simulink model "verify_Radiator_basic_mdl"  (R2016b)
settings: Solver=ode45  StartTime=0.0  StopTime=4800  MaxStep=100  RelTol=1e-3  EnableMultiTasking=on
undefined symbols (not defined in the file or in its folder): heat_capacity
libraries: carnot x2, simulink x1
settings Model: Creator=drhf  LastModifiedBy=drhf
settings DataIOCC: LimitDataPoints=on  SaveFormat=Array  SignalLoggingSaveFormat=ModelDataLogs
settings OptimizationCC: ExpressionDepthLimit=2147483647  LifeSpan=inf
settings DebuggingCC: UnderspecifiedInitializationDetection=Classic  MergeDetectMultiDrivingBlocksExec=none  SolverPrmCheckMsg=warning  FcnCallInpInsideContextMsg=warning  StateNameClashWarn=warning  SFUnexpectedBacktrackingDiag=warning  SFNoUnconditionalDefaultTransitionDiag=warning  SFExecutionAtInitializationDiag=none
settings HardwareCC: ProdBitPerPointer=32  ProdBitPerSizeT=32  ProdBitPerPtrDiffT=32  ProdLargestAtomicFloat=None  ProdIntDivRoundTo=Undefined  ProdEndianess=Unspecified  ProdWordSize=32  ProdHWDeviceType=32-bit Generic
settings ModelReferenceCC: PropagateSignalLabelsOutOfModel=off
settings GRTTargetCC: TargetLangStandard=C89/C90 (ANSI)  GeneratePreprocessorConditionals=Disable all  CombineOutputUpdateFcns=off  GRTInterface=on
settings ConfigComp: CovMetricSettings=dw  CovHtmlReporting=on  CovSaveCumulativeToWorkspaceVar=on  CovSaveSingleToWorkspaceVar=on  CovExternalEMLEnable=off

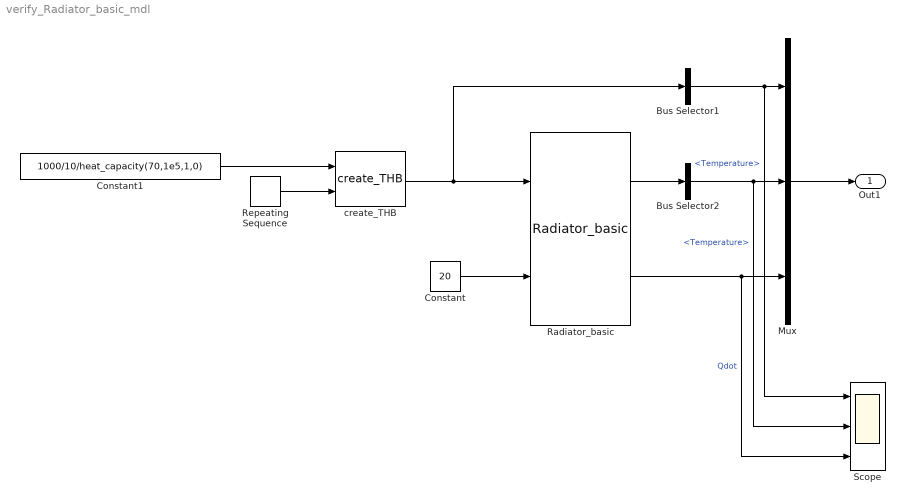
== system verify_Radiator_basic_mdl ==
  Bus Selector1 : BusSelector  OutputSignals=Temperature
  Bus Selector2 : BusSelector  OutputSignals=Temperature
  Constant : Constant  Value=20
  Constant1 : Constant  Value=1000/10/heat_capacity(70,1e5,1,0)
  Mux : Mux  Inputs=3
  Radiator_basic : carnot/Basic/Thermal_Models/Radiator_basic  pnomEN=1000  dtnomEN=50  expo=1.3  mcp=4182*1  tini=20
  Repeating Sequence : simulink/Sources/Repeating Sequence  rep_seq_t=[0 2 2.1 4 4.1 6 6.1 8.1]*60*10  rep_seq_y=[45 45 55 55 65 65 75 75]
  Scope : Scope  NumInputPorts=3
  create_THB : carnot/Source/Simple/create_THB  p=1e5  fluid=Water  mix=0  mix2=0  mix3=0  dia=0  hgt=0  mID=No Pressure Drop
  Out1 : Outport
  wires:
  Constant/1 -> Radiator_basic/2
  Radiator_basic/1 -> Bus Selector2/1
  Bus Selector2/1 -> Scope/2, Mux/2  "<Temperature>"
  Radiator_basic/2 -> Scope/3, Mux/3  "Qdot"
  create_THB/1 -> Radiator_basic/1, Bus Selector1/1
  Repeating Sequence/1 -> create_THB/2
  Bus Selector1/1 -> Scope/1, Mux/1  "<Temperature>"
  Mux/1 -> Out1/1
  Constant1/1 -> create_THB/1
